simulink library "SG_library"  (R2020a)
settings: Solver=VariableStepAuto  StartTime=0.0  StopTime=10.0  RelTol=1e-3
undefined symbols (not defined in the file): a, b, c, IO334, IO334_IO_FPGA, IO334_IO_src, IO334_SOS_FPGA, IO334_SOS_src, IO397, IO397_IO_FPGA, IO397_IO_src, IO397_SOS_FPGA, IO397_SOS_src
libraries: speedgoatlib_hdlCoder_IO3xx x35, $bdroot x20, xpcutilitieslib x8, hdlsllib x5, simulink x4, simulink_extras x1
(part 2 of 2)

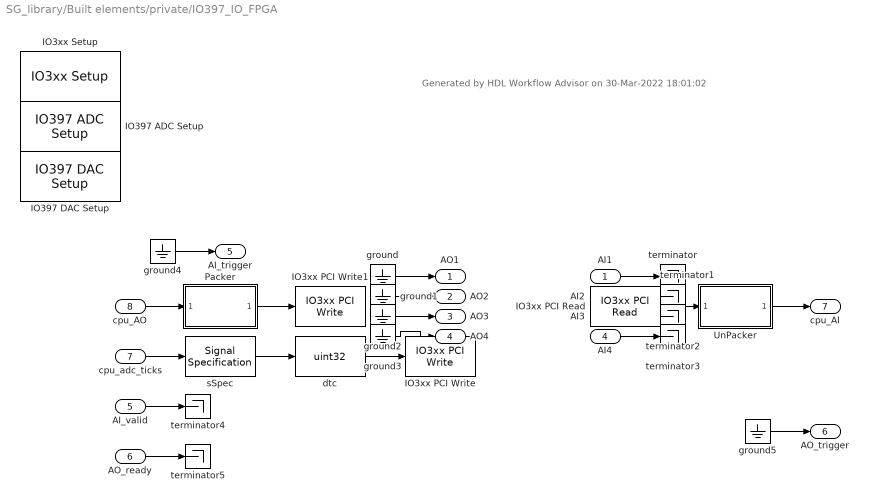
== system SG_library/Built elements/private/IO397_IO_FPGA ==
  note: Generated by HDL Workflow Advisor on 30-Mar-2022 18:01:02
  AI1 : Inport
  AI2 : Inport  Port=2
  AI3 : Inport  Port=3
  AI4 : Inport  Port=4
  AI_valid : Inport  Port=5
  AO_ready : Inport  Port=6
  cpu_adc_ticks : Inport  Port=7
  cpu_AO : Inport  Port=8
  IO397 ADC Setup : speedgoatlib_hdlCoder_IO3xx/IO397 ADC Setup  module_id=module_id  range1=+-10 V  range2=+-10 V  range3=+-10 V  range4=+-10 V
  IO397 DAC Setup : speedgoatlib_hdlCoder_IO3xx/IO397 DAC Setup  module_id=module_id  span=+-10 V
  IO3xx PCI Read : speedgoatlib_hdlCoder_IO3xx/IO3xx PCI Read  device_id=deviceIdx  module_id=module_id  board_type=IO3xx  port_name=cpu_AI  port_offset=hex2dec('118')  port_type=uint32  port_dim=2  strobe=hex2dec('120')  sample_time=ts
  IO3xx PCI Write : speedgoatlib_hdlCoder_IO3xx/IO3xx PCI Write  device_id=deviceIdx  module_id=module_id  board_type=IO3xx  port_name=cpu_adc_ticks  port_offset=hex2dec('100')  port_type=uint32  port_dim=1  strobe=0  sample_time=ts
  IO3xx PCI Write1 : speedgoatlib_hdlCoder_IO3xx/IO3xx PCI Write  device_id=deviceIdx  module_id=module_id  board_type=IO3xx  port_name=cpu_AO  port_offset=hex2dec('108')  port_type=uint32  port_dim=2  strobe=hex2dec('110')  sample_time=ts
  IO3xx Setup : speedgoatlib_hdlCoder_IO3xx/IO3xx Setup  mdl_ss_name=IO397_IO_src/IO397_IO_FPGA  board_type=IO397-50k  fpga_sync_mode=on  reset_mode=on  device_id=deviceIdx  module_id=module_id  pci_slot=slot  fpga_mat_file=C:\Speedgoat\Build\IO397_IO\hdlsrc\IO397_IO_src\IO397_IO_FPGA.mat  timestamp_mcs=03/30/22 18:00:22  timestamp=2203301755  tsreg=hex2dec('8')  bsf_file=IO397_IO_FPGA_2203301755.mcs  mcs=0
  Packer : Subsystem
  UnPacker : Subsystem
  dtc : DataTypeConversion  OutDataTypeStr=uint32  ConvertRealWorld=Stored Integer (SI)  RndMeth=Zero
  ground{,1..5} (6 alike) : Ground
  sSpec : SignalSpecification  OutDataTypeStr=fixdt(0,32,0)
  terminator{,1..5} (6 alike) : Terminator
  AO1 : Outport  VectorParamsAs1DForOutWhenUnconnected=off
  AO2 : Outport  Port=2  VectorParamsAs1DForOutWhenUnconnected=off
  AO3 : Outport  Port=3  VectorParamsAs1DForOutWhenUnconnected=off
  AO4 : Outport  Port=4  VectorParamsAs1DForOutWhenUnconnected=off
  AI_trigger : Outport  Port=5  VectorParamsAs1DForOutWhenUnconnected=off
  AO_trigger : Outport  Port=6  VectorParamsAs1DForOutWhenUnconnected=off
  cpu_AI : Outport  Port=7  VectorParamsAs1DForOutWhenUnconnected=off
  wires:
  IO3xx PCI Read/1 -> UnPacker/1(packed)
  UnPacker/1(unpacked) -> cpu_AI/1
  ground5/1 -> AO_trigger/1
  ground4/1 -> AI_trigger/1
  ground3/1 -> AO4/1
  ground2/1 -> AO3/1
  ground1/1 -> AO2/1
  ground/1 -> AO1/1
  Packer/1(packed) -> IO3xx PCI Write1/1
  cpu_AO/1 -> Packer/1(unpacked)
  dtc/1 -> IO3xx PCI Write/1
  sSpec/1 -> dtc/1
  cpu_adc_ticks/1 -> sSpec/1
  AO_ready/1 -> terminator5/1
  AI_valid/1 -> terminator4/1
  AI4/1 -> terminator3/1
  AI3/1 -> terminator2/1
  AI2/1 -> terminator1/1
  AI1/1 -> terminator/1

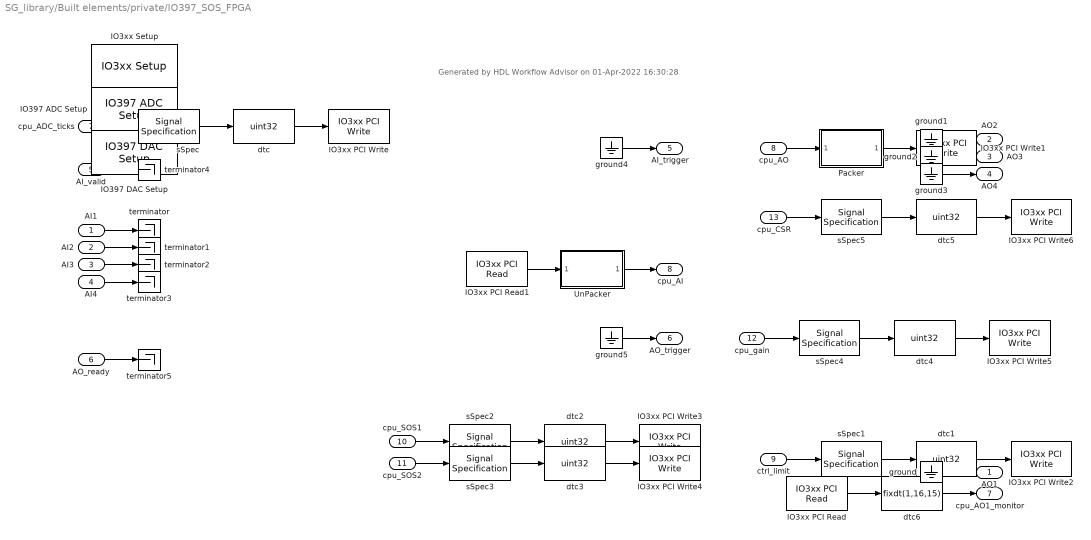
== system SG_library/Built elements/private/IO397_SOS_FPGA ==
  note: Generated by HDL Workflow Advisor on 01-Apr-2022 16:30:28
  AI1 : Inport
  AI2 : Inport  Port=2
  AI3 : Inport  Port=3
  AI4 : Inport  Port=4
  AI_valid : Inport  Port=5
  AO_ready : Inport  Port=6
  cpu_ADC_ticks : Inport  Port=7
  cpu_AO : Inport  Port=8
  ctrl_limit : Inport  Port=9
  cpu_SOS1 : Inport  Port=10
  cpu_SOS2 : Inport  Port=11
  cpu_gain : Inport  Port=12
  cpu_CSR : Inport  Port=13
  IO397 ADC Setup : speedgoatlib_hdlCoder_IO3xx/IO397 ADC Setup  module_id=module_id  range1=+-10 V  range2=+-10 V  range3=+-10 V  range4=+-10 V
  IO397 DAC Setup : speedgoatlib_hdlCoder_IO3xx/IO397 DAC Setup  module_id=module_id  span=+-10 V
  IO3xx PCI Read : speedgoatlib_hdlCoder_IO3xx/IO3xx PCI Read  device_id=deviceIdx  module_id=module_id  board_type=IO3xx  port_name=cpu_AO1_monitor  port_offset=hex2dec('124')  port_type=uint32  port_dim=1  strobe=0  sample_time=ts
  IO3xx PCI Read1 : speedgoatlib_hdlCoder_IO3xx/IO3xx PCI Read  device_id=deviceIdx  module_id=module_id  board_type=IO3xx  port_name=cpu_AI  port_offset=hex2dec('128')  port_type=uint32  port_dim=2  strobe=hex2dec('130')  sample_time=ts
  IO3xx PCI Write : speedgoatlib_hdlCoder_IO3xx/IO3xx PCI Write  device_id=deviceIdx  module_id=module_id  board_type=IO3xx  port_name=cpu_ADC_ticks  port_offset=hex2dec('100')  port_type=uint32  port_dim=1  strobe=0  sample_time=ts
  IO3xx PCI Write1 : speedgoatlib_hdlCoder_IO3xx/IO3xx PCI Write  device_id=deviceIdx  module_id=module_id  board_type=IO3xx  port_name=cpu_AO  port_offset=hex2dec('108')  port_type=uint32  port_dim=2  strobe=hex2dec('110')  sample_time=ts
  IO3xx PCI Write2 : speedgoatlib_hdlCoder_IO3xx/IO3xx PCI Write  device_id=deviceIdx  module_id=module_id  board_type=IO3xx  port_name=ctrl_limit  port_offset=hex2dec('104')  port_type=uint32  port_dim=1  strobe=0  sample_time=ts
  IO3xx PCI Write3 : speedgoatlib_hdlCoder_IO3xx/IO3xx PCI Write  device_id=deviceIdx  module_id=module_id  board_type=IO3xx  port_name=cpu_SOS1  port_offset=hex2dec('180')  port_type=uint32  port_dim=24  strobe=hex2dec('200')  sample_time=ts
  IO3xx PCI Write4 : speedgoatlib_hdlCoder_IO3xx/IO3xx PCI Write  device_id=deviceIdx  module_id=module_id  board_type=IO3xx  port_name=cpu_SOS2  port_offset=hex2dec('280')  port_type=uint32  port_dim=24  strobe=hex2dec('300')  sample_time=ts
  IO3xx PCI Write5 : speedgoatlib_hdlCoder_IO3xx/IO3xx PCI Write  device_id=deviceIdx  module_id=module_id  board_type=IO3xx  port_name=cpu_gain  port_offset=hex2dec('118')  port_type=uint32  port_dim=2  strobe=hex2dec('120')  sample_time=ts
  IO3xx PCI Write6 : speedgoatlib_hdlCoder_IO3xx/IO3xx PCI Write  device_id=deviceIdx  module_id=module_id  board_type=IO3xx  port_name=cpu_CSR  port_offset=hex2dec('114')  port_type=uint32  port_dim=1  strobe=0  sample_time=ts
  IO3xx Setup : speedgoatlib_hdlCoder_IO3xx/IO3xx Setup  mdl_ss_name=IO397_SOS_src/IO397_SOS_FPGA  board_type=IO397-50k  fpga_sync_mode=on  reset_mode=on  device_id=deviceIdx  module_id=module_id  pci_slot=slot  fpga_mat_file=C:\Speedgoat\Build\IO397_SOS\hdlsrc\IO397_SOS_src\IO397_SOS_FPGA.mat  timestamp_mcs=04/01/22 16:29:43  timestamp=2204011623  tsreg=hex2dec('8')  bsf_file=IO397_SOS_FPGA_2204011623.mcs  mcs=0
  Packer : Subsystem
  UnPacker : Subsystem
  dtc{,1..5} (6 alike) : DataTypeConversion  OutDataTypeStr=uint32  ConvertRealWorld=Stored Integer (SI)  RndMeth=Zero
  dtc6 : DataTypeConversion  OutDataTypeStr=fixdt(1,16,15)  ConvertRealWorld=Stored Integer (SI)  RndMeth=Zero
  ground{,1..5} (6 alike) : Ground
  sSpec : SignalSpecification  OutDataTypeStr=fixdt(0,32,0)
  sSpec1 : SignalSpecification  OutDataTypeStr=fixdt(1,16,15)
  sSpec2 : SignalSpecification  OutDataTypeStr=fixdt(1,32,20)
  sSpec3 : SignalSpecification  OutDataTypeStr=fixdt(1,32,20)
  sSpec4 : SignalSpecification  OutDataTypeStr=fixdt(1,32,20)
  sSpec5 : SignalSpecification  OutDataTypeStr=fixdt(0,8,0)
  terminator{,1..5} (6 alike) : Terminator
  AO1 : Outport  VectorParamsAs1DForOutWhenUnconnected=off
  AO2 : Outport  Port=2  VectorParamsAs1DForOutWhenUnconnected=off
  AO3 : Outport  Port=3  VectorParamsAs1DForOutWhenUnconnected=off
  AO4 : Outport  Port=4  VectorParamsAs1DForOutWhenUnconnected=off
  AI_trigger : Outport  Port=5  VectorParamsAs1DForOutWhenUnconnected=off
  AO_trigger : Outport  Port=6  VectorParamsAs1DForOutWhenUnconnected=off
  cpu_AO1_monitor : Outport  Port=7  VectorParamsAs1DForOutWhenUnconnected=off
  cpu_AI : Outport  Port=8  VectorParamsAs1DForOutWhenUnconnected=off
  wires:
  IO3xx PCI Read1/1 -> UnPacker/1(packed)
  UnPacker/1(unpacked) -> cpu_AI/1
  IO3xx PCI Read/1 -> dtc6/1
  dtc6/1 -> cpu_AO1_monitor/1
  ground5/1 -> AO_trigger/1
  ground4/1 -> AI_trigger/1
  ground3/1 -> AO4/1
  ground2/1 -> AO3/1
  ground1/1 -> AO2/1
  ground/1 -> AO1/1
  dtc5/1 -> IO3xx PCI Write6/1
  sSpec5/1 -> dtc5/1
  cpu_CSR/1 -> sSpec5/1
  dtc4/1 -> IO3xx PCI Write5/1
  sSpec4/1 -> dtc4/1
  cpu_gain/1 -> sSpec4/1
  dtc3/1 -> IO3xx PCI Write4/1
  sSpec3/1 -> dtc3/1
  cpu_SOS2/1 -> sSpec3/1
  dtc2/1 -> IO3xx PCI Write3/1
  sSpec2/1 -> dtc2/1
  cpu_SOS1/1 -> sSpec2/1
  dtc1/1 -> IO3xx PCI Write2/1
  sSpec1/1 -> dtc1/1
  ctrl_limit/1 -> sSpec1/1
  Packer/1(packed) -> IO3xx PCI Write1/1
  cpu_AO/1 -> Packer/1(unpacked)
  dtc/1 -> IO3xx PCI Write/1
  sSpec/1 -> dtc/1
  cpu_ADC_ticks/1 -> sSpec/1
  AO_ready/1 -> terminator5/1
  AI_valid/1 -> terminator4/1
  AI4/1 -> terminator3/1
  AI3/1 -> terminator2/1
  AI2/1 -> terminator1/1
  AI1/1 -> terminator/1

== system SG_library/Source elements/Discrete SOS section DFII serial/Subsystem2 ==
  trigger : Inport
  Bit Shift : hdlsllib/Logic and Bit Operations/Bit Shift  mode=Shift Right Logical  N=1
  Compare To Constant1 : simulink/Logic and Bit Operations/Compare To Constant  relop===  const=8  OutDataTypeStr=boolean
  Delay1 : Delay  DelayLength=1  ExternalReset=Level hold
      settings: InputPortMap=u0,r5
  HDL Counter1 : hdlsllib/Sources/HDL Counter  CountType=Free running  CountInit=0  CountStep=1  CountMax=4  CountFromType=Initial value  CountFrom=0  CountResetPort=on  CountLoadPort=off  CountEnbPort=on  CountDirPort=off  CountDataType=Unsigned  CountWordLen=4  CountFracLen=0  CountSampTime=-1
  NOT : Logic  Operator=NOT  IconShape=distinctive  AllPortsSameDT=off  OutDataTypeStr=boolean
  OR : Logic  Operator=OR  IconShape=distinctive  AllPortsSameDT=off  OutDataTypeStr=boolean
  count : Outport
  wires:
  Compare To Constant1/1 -> Delay1/2
  HDL Counter1/1 -> Bit Shift/1, Compare To Constant1/1
  NOT/1 -> HDL Counter1/1
  OR/1 -> NOT/1, Delay1/1, HDL Counter1/2
  trigger/1 -> OR/1
  Delay1/1 -> OR/2
  Bit Shift/1 -> count/1

== system SG_library/Built elements/private/IO334_IO_FPGA/Packer ==
  unpacked : Inport
  pack : xpcutilitieslib/Bit Packing   MaskBitPatterns={[0:15 16:31 32:47 48:63 64:79 80:95 96:111 112:127 128:143 144:159 160:175 176:191 192:207 208:223 224:239 240:255 ]}  MaskPackDataType=uint32  MaskPackDataSize=8
      settings: SourceProductBaseCode=XP
  sSpec : SignalSpecification  OutDataTypeStr=fixdt(1,16,15)
  upconvert : DataTypeConversion  OutDataTypeStr=uint16  ConvertRealWorld=Stored Integer (SI)  RndMeth=Zero
  packed : Outport
  wires:
  pack/1 -> packed/1
  upconvert/1 -> pack/1
  sSpec/1 -> upconvert/1
  unpacked/1 -> sSpec/1

== system SG_library/Built elements/private/IO334_IO_FPGA/UnPacker ==
  packed : Inport
  downconvert : DataTypeConversion  OutDataTypeStr=fixdt(1,16,15)  ConvertRealWorld=Stored Integer (SI)  RndMeth=Zero
  unpack : xpcutilitieslib/Bit Unpacking   SignExtend=on  MaskBitPatterns={[0:15 16:31 32:47 48:63 64:79 80:95 96:111 112:127 128:143 144:159 160:175 176:191 192:207 208:223 224:239 240:255 ]}  MaskPackDataType=uint32  MaskPackDataSize=8  MaskUnpackDataTypes={'uint16'}  MaskUnpackDataSizes={16}
      settings: SourceProductBaseCode=XP
  unpacked : Outport
  wires:
  downconvert/1 -> unpacked/1
  unpack/1 -> downconvert/1
  packed/1 -> unpack/1

== system SG_library/Built elements/private/IO334_SOS_FPGA/Packer ==
  unpacked : Inport
  pack : xpcutilitieslib/Bit Packing   MaskBitPatterns={[0:15 16:31 32:47 48:63 64:79 80:95 96:111 112:127 128:143 144:159 160:175 176:191 192:207 208:223 224:239 240:255 ]}  MaskPackDataType=uint32  MaskPackDataSize=8
      settings: SourceProductBaseCode=XP
  sSpec : SignalSpecification  OutDataTypeStr=fixdt(1,16,15)
  upconvert : DataTypeConversion  OutDataTypeStr=uint16  ConvertRealWorld=Stored Integer (SI)  RndMeth=Zero
  packed : Outport
  wires:
  pack/1 -> packed/1
  upconvert/1 -> pack/1
  sSpec/1 -> upconvert/1
  unpacked/1 -> sSpec/1

== system SG_library/Built elements/private/IO334_SOS_FPGA/UnPacker ==
  packed : Inport
  downconvert : DataTypeConversion  OutDataTypeStr=fixdt(1,16,15)  ConvertRealWorld=Stored Integer (SI)  RndMeth=Zero
  unpack : xpcutilitieslib/Bit Unpacking   SignExtend=on  MaskBitPatterns={[0:15 16:31 32:47 48:63 64:79 80:95 96:111 112:127 128:143 144:159 160:175 176:191 192:207 208:223 224:239 240:255 ]}  MaskPackDataType=uint32  MaskPackDataSize=8  MaskUnpackDataTypes={'uint16'}  MaskUnpackDataSizes={16}
      settings: SourceProductBaseCode=XP
  unpacked : Outport
  wires:
  downconvert/1 -> unpacked/1
  unpack/1 -> downconvert/1
  packed/1 -> unpack/1

== system SG_library/Built elements/private/IO397_IO_FPGA/Packer ==
  unpacked : Inport
  pack : xpcutilitieslib/Bit Packing   MaskBitPatterns={[0:15 16:31 32:47 48:63 ]}  MaskPackDataType=uint32  MaskPackDataSize=2
      settings: SourceProductBaseCode=XP
  sSpec : SignalSpecification  OutDataTypeStr=fixdt(1,16,15)
  upconvert : DataTypeConversion  OutDataTypeStr=uint16  ConvertRealWorld=Stored Integer (SI)  RndMeth=Zero
  packed : Outport
  wires:
  pack/1 -> packed/1
  upconvert/1 -> pack/1
  sSpec/1 -> upconvert/1
  unpacked/1 -> sSpec/1

== system SG_library/Built elements/private/IO397_IO_FPGA/UnPacker ==
  packed : Inport
  downconvert : DataTypeConversion  OutDataTypeStr=fixdt(1,16,15)  ConvertRealWorld=Stored Integer (SI)  RndMeth=Zero
  unpack : xpcutilitieslib/Bit Unpacking   SignExtend=on  MaskBitPatterns={[0:15 16:31 32:47 48:63 ]}  MaskPackDataType=uint32  MaskPackDataSize=2  MaskUnpackDataTypes={'uint16'}  MaskUnpackDataSizes={4}
      settings: SourceProductBaseCode=XP
  unpacked : Outport
  wires:
  downconvert/1 -> unpacked/1
  unpack/1 -> downconvert/1
  packed/1 -> unpack/1

== system SG_library/Built elements/private/IO397_SOS_FPGA/Packer ==
  unpacked : Inport
  pack : xpcutilitieslib/Bit Packing   MaskBitPatterns={[0:15 16:31 32:47 48:63 ]}  MaskPackDataType=uint32  MaskPackDataSize=2
      settings: SourceProductBaseCode=XP
  sSpec : SignalSpecification  OutDataTypeStr=fixdt(1,16,15)
  upconvert : DataTypeConversion  OutDataTypeStr=uint16  ConvertRealWorld=Stored Integer (SI)  RndMeth=Zero
  packed : Outport
  wires:
  pack/1 -> packed/1
  upconvert/1 -> pack/1
  sSpec/1 -> upconvert/1
  unpacked/1 -> sSpec/1

== system SG_library/Built elements/private/IO397_SOS_FPGA/UnPacker ==
  packed : Inport
  downconvert : DataTypeConversion  OutDataTypeStr=fixdt(1,16,15)  ConvertRealWorld=Stored Integer (SI)  RndMeth=Zero
  unpack : xpcutilitieslib/Bit Unpacking   SignExtend=on  MaskBitPatterns={[0:15 16:31 32:47 48:63 ]}  MaskPackDataType=uint32  MaskPackDataSize=2  MaskUnpackDataTypes={'uint16'}  MaskUnpackDataSizes={4}
      settings: SourceProductBaseCode=XP
  unpacked : Outport
  wires:
  downconvert/1 -> unpacked/1
  unpack/1 -> downconvert/1
  packed/1 -> unpack/1

== matlab function SG_library/Built elements/IO397_SOS/MATLAB Function ==
  data: rst input; csr output; ctrl_on input
function csr = f(rst, ctrl_on)
    csr = bitor(uint8(rst), bitshift(uint8(ctrl_on), 1));
end

== matlab function SG_library/Source elements/Discrete SOS section DFII serial/MATLAB Function ==
  data: sos input; u input; a output size=1; x input size=2; idx input size=1; fb input size=1; cntr input size=1; b output size=1; c output size=1
function [a, b, c] = serializer(sos, u, x, idx, fb, cntr)
    N = 4;
    switch cntr
        case 0
            a = x(2);
            b = -sos(idx + 5*N); % a2
            c = u;
        case 1
            a = x(1);
            b = -sos(idx + 4*N); % a1
            c = fb;
        case 2
            a = fb;
            b = sos(idx); % b0
            c = zeros(1, 'like', u);
        case 3
            a = x(1);
            b = sos(idx + N); % b1
            c = fb;
        otherwise
            a = x(2);
            b = sos(idx + 2*N); % b2
            c = fb;
    end
end

== matlab function SG_library/Built elements/IO397_SOS/MATLAB Function1 ==
  data: range1 input; gains output; range2 input; span input
function gains = fcn(range1, range2, span)
    gains = [0 0];
    switch range1
        case 1
            gains(1) = 5.12;
        case 2
            gains(1) = 10;
        case 3
            gains(1) = 10.24;
        case 4
            gains(1) = 10;
        case 5
            gains(1) = 10.24;
        case 6
            gains(1) = 20;
        case 7
            gains(1) = 20.48;
        otherwise
            error('invalid case');
    end
    
    switch range2
        case 1
            gains(2) = 5.12;
        case 2
            gains(2) = 10;
        case 3
            gains(2) = 10.24;
        case 4
            gains(2) = 10;
        case 5
            gains(2) = 10.24;
        case 6
            gains(2) = 20;
        case 7
            gains(2) = 20.48;
        otherwise
            error('invalid case');
    end
    
    switch span
        case 1
            gains = gains/5;
        case {2, 3}
            gains = gains/10;
        case 4
            gains = gains/20;
        otherwise
            error('invalid case');
    end
    
    
end
